simulink model "sampleModel1488"  (R2023a)
settings: Solver=VariableStepAuto  StartTime=0.0  StopTime=10.0  RelTol=1e-3
undefined symbols (not defined in the file): b011101a, b0c8, bf87616c, DiscIntNeverNeededParam, Newton, Raphson
libraries: simulink x171, slpidlib x32, simulink_need_slupdate x2
(part 5 of 6)

== system sampleModel1488/cfblk153/cfblk12 ==
  cfblk1 : Inport
  cfblk9 : Inport  Port=2
  cfblk11 : Delay  SampleTime=1
  cfblk12 : Delay  SampleTime=1
  cfblk3 : DiscreteFilter  SampleTime=1
  cfblk4 : Gain  Gain=[185491925.881963]
  cfblk5 : Product
  cfblk6 : ComplexToMagnitudeAngle
  cfblk7 : MinMax  Inputs=3
  cfblk8 : simulink/Math Operations/Slider Gain  gain=1  low=0  high=2
  cfblk2 : Outport
  cfblk10 : Outport  Port=2
  wires:
  cfblk9/1 -> cfblk8/1
  cfblk3/1 -> cfblk6/1
  cfblk7/1 -> cfblk2/1, cfblk3/1
  cfblk8/1 -> cfblk4/1
  cfblk5/1 -> cfblk7/2
  cfblk1/1 -> cfblk5/1, cfblk7/3
  cfblk4/1 -> cfblk10/1
  cfblk6/1 -> cfblk11/1
  cfblk11/1 -> cfblk7/1
  cfblk6/2 -> cfblk12/1
  cfblk12/1 -> cfblk5/2

== system sampleModel1488/cfblk153/cfblk8 ==
  cfblk1 : Inport
  cfblk9 : Inport  Port=2
  cfblk3 : DiscreteTransferFcn  SampleTime=1
  cfblk4 : simulink/Discrete/Transfer Fcn First Order  PoleZ=0.95  ICPrevOutput=0.0  DoSatur=off
  cfblk5 : simulink/Discrete/Transfer Fcn Lead or Lag  PoleZ=0.95  ZeroZ=0.75  ICPrevOutput=0.0  ICPrevInput=0.0  DoSatur=off
  cfblk6 : ComplexToRealImag
  cfblk7 : Product  Inputs=**
  cfblk8 : Constant  Value=[-545162540.511820]  SampleTime=1
  cfblk2 : Outport
  cfblk10 : Outport  Port=2
  wires:
  cfblk1/1 -> cfblk5/1
  cfblk5/1 -> cfblk2/1
  cfblk7/1 -> cfblk4/1
  cfblk3/1 -> cfblk6/1
  cfblk6/1 -> cfblk7/1
  cfblk8/1 -> cfblk7/2
  cfblk9/1 -> cfblk3/1
  cfblk4/1 -> cfblk10/1

== system sampleModel1488/cfblk153/cfblk9 ==
  cfblk1 : Inport
  cfblk7 : Inport  Port=2
  cfblk3 : DiscreteZeroPole  Poles=[0 0.5]  Gain=1
  cfblk4 : Bias  Bias=[67062085.652409]  SaturateOnIntegerOverflow=off
  cfblk5 : ComplexToRealImag
  cfblk6 : Rounding
  cfblk9 : Delay  SampleTime=1
  cfblk2 : Outport
  cfblk8 : Outport  Port=2
  wires:
  cfblk3/1 -> cfblk6/1
  cfblk5/1 -> cfblk8/1
  cfblk5/2 -> cfblk2/1
  cfblk1/1 -> cfblk5/1
  cfblk7/1 -> cfblk4/1
  cfblk6/1 -> cfblk9/1
  cfblk9/1 -> cfblk3/1

== system sampleModel1488/cfblk154/cfblk7 ==
  cfblk1 : Inport
  cfblk6 : Inport  Port=2
  cfblk3 : Delay  ShowEnablePort=on  SampleTime=1
      settings: InputPortMap=u0,e6
  cfblk4 : simulink/Discrete/Difference  ICPrevInput=0.0  OutMin=[]  OutMax=[]  OutDataTypeStr=Inherit: Inherit via back propagation  OutDataType=fixdt(1, 16)  OutScaling=2^-10  DoSatur=off
  cfblk5 : Rounding
  cfblk2 : Outport
  cfblk7 : Outport  Port=2
  wires:
  cfblk3/1 -> cfblk7/1
  cfblk1/1 -> cfblk2/1
  cfblk4/1 -> cfblk3/1
  cfblk6/1 -> cfblk5/1, cfblk3/2
  cfblk5/1 -> cfblk4/1

== system sampleModel1488/cfblk155/cfblk5 ==
  cfblk1 : Inport
  cfblk12 : Inport  Port=2
  cfblk13 : Inport  Port=3
  cfblk14 : Inport  Port=4
  cfblk10 : Constant  Value=[300138344.882590]  SampleTime=1
  cfblk11 : Constant  Value=[340060627.789807]  SampleTime=1
  cfblk3 : DiscreteIntegrator  ICPrevOutput=DiscIntNeverNeededParam  ICPrevScaledInput=DiscIntNeverNeededParam
  cfblk4 : DiscreteFilter  SampleTime=1
  cfblk5 : simulink/Discrete/Tapped Delay  vinit=0.0  samptime=-1  NumDelays=1  DelayOrder=Oldest  includeCurrent=off
  cfblk6 : UnaryMinus
  cfblk7 : DotProduct  OutDataTypeStr=Inherit: Inherit via internal rule
  cfblk8 : DotProduct  OutDataTypeStr=Inherit: Inherit via internal rule
  cfblk9 : Squeeze
  cfblk2 : Outport
  cfblk15 : Outport  Port=2
  wires:
  cfblk8/1 -> cfblk3/1
  cfblk4/1 -> cfblk2/1
  cfblk10/1 -> cfblk7/1
  cfblk3/1 -> cfblk7/2
  cfblk5/1 -> cfblk8/1
  cfblk1/1 -> cfblk5/1
  cfblk11/1 -> cfblk6/1
  cfblk14/1 -> cfblk9/1
  cfblk13/1 -> cfblk8/2
  cfblk9/1 -> cfblk4/1
  cfblk7/1 -> cfblk15/1

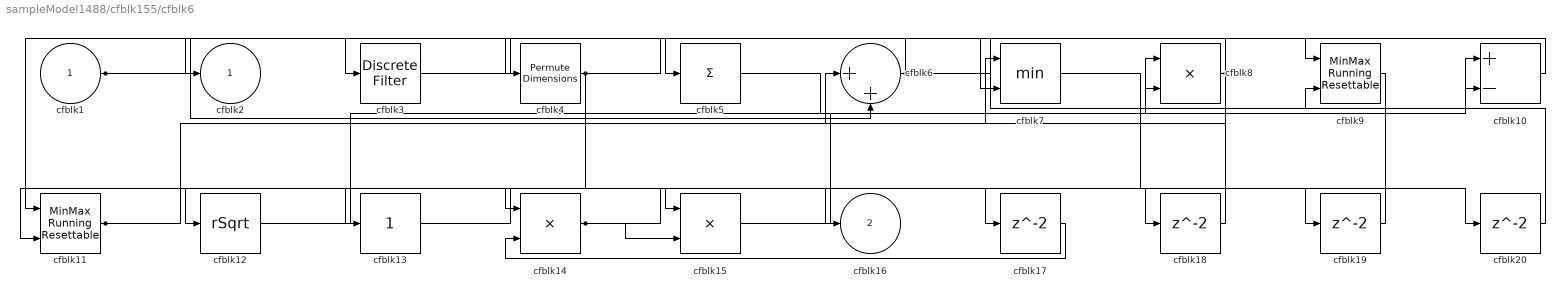
== system sampleModel1488/cfblk155/cfblk6 ==
  cfblk1 : Inport
  cfblk10 : Sum  Inputs=+-
  cfblk11 : simulink/Math Operations/MinMax Running Resettable  Function=min  vinit=0.0
  cfblk12 : Sqrt  Operator=rSqrt  AlgorithmType=Newton-Raphson
  cfblk13 : simulink/Math Operations/Slider Gain  gain=1  low=0  high=2
  cfblk14 : Product
  cfblk15 : Product  Inputs=**
  cfblk{17..20} (4 alike) : Delay  SampleTime=1
  cfblk3 : DiscreteFilter  SampleTime=1
  cfblk4 : PermuteDimensions
  cfblk5 : Sum  Inputs=+
  cfblk6 : Sum  Inputs=|++
  cfblk7 : MinMax  Inputs=2
  cfblk8 : Product
  cfblk9 : simulink/Math Operations/MinMax Running Resettable  Function=min  vinit=0.0
  cfblk2 : Outport
  cfblk16 : Outport  Port=2
  wires:
  cfblk4/1 -> cfblk12/1, cfblk7/2
  cfblk10/1 -> cfblk11/1
  cfblk3/1 -> cfblk5/1
  cfblk15/1 -> cfblk8/1
  cfblk11/1 -> cfblk7/1, cfblk13/1, cfblk18/1
  cfblk13/1 -> cfblk16/1
  cfblk12/1 -> cfblk10/1
  cfblk9/1 -> cfblk14/1
  cfblk5/1 -> cfblk8/2
  cfblk6/1 -> cfblk9/1, cfblk3/1, cfblk10/2
  cfblk8/1 -> cfblk11/2, cfblk2/1, cfblk17/1
  cfblk14/1 -> cfblk15/2, cfblk20/1
  cfblk1/1 -> cfblk6/2, cfblk4/1
  cfblk17/1 -> cfblk14/2
  cfblk18/1 -> cfblk6/1
  cfblk7/1 -> cfblk19/1
  cfblk19/1 -> cfblk15/1
  cfblk20/1 -> cfblk9/2

== system sampleModel1488/cfblk156/cfblk10 ==
  cfblk1 : Inport
  cfblk10 : Inport  Port=2
  cfblk11 : Inport  Port=3
  cfblk12 : Inport  Port=4
  cfblk13 : Inport  Port=5
  cfblk14 : Inport  Port=6
  cfblk15 : Inport  Port=7
  cfblk3 : simulink/Discrete/Transfer Fcn Real Zero  ZeroZ=0.75  ICPrevInput=0.0  DoSatur=off
  cfblk4 : Delay  DelayLengthSource=Input port  SampleTime=1
      settings: InputPortMap=u0,p1
  cfblk5 : simulink/Math Operations/MinMax Running Resettable  Function=min  vinit=0.0
  cfblk6 : UnaryMinus
  cfblk7 : Squeeze
  cfblk8 : Rounding
  cfblk9 : Constant  Value=[895322643.811582]  SampleTime=1
  cfblk2 : Outport
  wires:
  cfblk10/1 -> cfblk4/1
  cfblk5/1 -> cfblk2/1
  cfblk3/1 -> cfblk6/1
  cfblk1/1 -> cfblk5/1
  cfblk13/1 -> cfblk4/2
  cfblk8/1 -> cfblk5/2
  cfblk7/1 -> cfblk8/1
  cfblk11/1 -> cfblk7/1
  cfblk15/1 -> cfblk3/1

== system sampleModel1488/cfblk156/cfblk11 ==
  cfblk1 : Inport
  cfblk6 : Inport  Port=2
  cfblk7 : Inport  Port=3
  cfblk8 : Inport  Port=4
  cfblk9 : Inport  Port=5
  cfblk3 : Product  Inputs=*
  cfblk4 : Squeeze
  cfblk5 : Constant  Value=[-712808178.157730]  SampleTime=1
  cfblk2 : Outport
  cfblk10 : Outport  Port=2
  wires:
  cfblk6/1 -> cfblk2/1
  cfblk1/1 -> cfblk4/1
  cfblk8/1 -> cfblk10/1
  cfblk4/1 -> cfblk3/1

== system sampleModel1488/cfblk156/cfblk12 ==
  cfblk1 : Inport
  cfblk9 : Inport  Port=2
  cfblk10 : Inport  Port=3
  cfblk11 : Inport  Port=4
  cfblk3 : simulink/Discrete/Transfer Fcn Lead or Lag  PoleZ=0.95  ZeroZ=0.75  ICPrevOutput=0.0  ICPrevInput=0.0  DoSatur=off
  cfblk4 : Bias  Bias=[-19724596.447759]  SaturateOnIntegerOverflow=off
  cfblk5 : Abs  SaturateOnIntegerOverflow=off
  cfblk6 : Product
  cfblk7 : Assignment  DiagnosticForDimensions=Warning  IndexOptions=Index vector (dialog)  Indices=1  OutputSizes=1
  cfblk8 : Constant  Value=[-371159435.516197]  SampleTime=1
  cfblk2 : Outport
  wires:
  cfblk6/1 -> cfblk7/1
  cfblk10/1 -> cfblk5/1
  cfblk9/1 -> cfblk3/1
  cfblk3/1 -> cfblk4/1
  cfblk4/1 -> cfblk6/1
  cfblk7/1 -> cfblk2/1
  cfblk11/1 -> cfblk6/2
  cfblk1/1 -> cfblk7/2

== system sampleModel1488/cfblk157/cfblk12 ==
  cfblk1 : Inport
  cfblk5 : Inport  Port=2
  cfblk6 : Inport  Port=3
  cfblk7 : Inport  Port=4
  cfblk8 : Inport  Port=5
  Action Port : ActionPort  ActionPortLabel=if(u1 >= 0)
  cfblk3 : Product
  cfblk4 : ComplexToMagnitudeAngle
  cfblk2 : Outport
  wires:
  cfblk5/1 -> cfblk4/1
  cfblk1/1 -> cfblk2/1
  cfblk6/1 -> cfblk3/1
  cfblk4/1 -> cfblk3/2

== system sampleModel1488/cfblk157/cfblk13 ==
  cfblk1 : Inport
  cfblk11 : Inport  Port=2
  cfblk12 : Inport  Port=3
  cfblk13 : Inport  Port=4
  Action Port : ActionPort  ActionPortLabel=else
  cfblk10 : Constant  Value=[-560694397.866348]  SampleTime=1
  cfblk3 : simulink/Discrete/Tapped Delay  vinit=0.0  samptime=-1  NumDelays=1  DelayOrder=Oldest  includeCurrent=off
  cfblk4 : simulink/Discrete/Transfer Fcn Real Zero  ZeroZ=0.75  ICPrevInput=0.0  DoSatur=off
  cfblk5 : UnaryMinus
  cfblk6 : Signum
  cfblk7 : Signum
  cfblk8 : Gain  Gain=[983882556.458164]
  cfblk9 : Constant  Value=[-401635952.431954]  SampleTime=1
  cfblk2 : Outport
  cfblk14 : Outport  Port=2
  cfblk15 : Outport  Port=3
  cfblk16 : Outport  Port=4
  wires:
  cfblk11/1 -> cfblk6/1
  cfblk10/1 -> cfblk5/1
  cfblk6/1 -> cfblk14/1
  cfblk7/1 -> cfblk8/1
  cfblk5/1 -> cfblk16/1
  cfblk13/1 -> cfblk7/1
  cfblk8/1 -> cfblk3/1
  cfblk1/1 -> cfblk2/1
  cfblk3/1 -> cfblk15/1
  cfblk12/1 -> cfblk4/1

== system sampleModel1488/cfblk158/cfblk11 ==
  cfblk1 : Inport
  cfblk15 : Inport  Port=2
  cfblk16 : Inport  Port=3
  cfblk17 : Inport  Port=4
  cfblk10 : UnaryMinus
  cfblk11 : Product  Inputs=*
  cfblk12 : Constant  Value=[-127465425.334475]  SampleTime=1
  cfblk13 : Constant  Value=[-255537626.018522]  SampleTime=1
  cfblk14 : Constant  Value=[421184774.119450]  SampleTime=1
  cfblk3 : DiscreteStateSpace
  cfblk4 : Abs  SaturateOnIntegerOverflow=off
  cfblk5 : Sum  Inputs=+
  cfblk6 : Squeeze
  cfblk7 : Product  Inputs=*
  cfblk8 : Bias  Bias=[52580442.536765]  SaturateOnIntegerOverflow=off
  cfblk9 : Sum  Inputs=|++
  cfblk2 : Outport
  wires:
  cfblk12/1 -> cfblk5/1
  cfblk16/1 -> cfblk11/1
  cfblk1/1 -> cfblk6/1
  cfblk14/1 -> cfblk9/1
  cfblk8/1 -> cfblk2/1
  cfblk6/1 -> cfblk4/1
  cfblk9/1 -> cfblk8/1
  cfblk13/1 -> cfblk10/1
  cfblk11/1 -> cfblk3/1
  cfblk10/1 -> cfblk9/2
  cfblk5/1 -> cfblk7/1

== system sampleModel1488/cfblk158/cfblk12 ==
  cfblk1 : Inport
  cfblk10 : Constant  Value=[-764079549.209031]  SampleTime=1
  cfblk11 : Delay  SampleTime=1
  cfblk12 : Delay  SampleTime=1
  cfblk3 : simulink/Discrete/Tapped Delay  vinit=0.0  samptime=-1  NumDelays=1  DelayOrder=Oldest  includeCurrent=off
  cfblk4 : DiscreteStateSpace
  cfblk5 : Sqrt  Operator=rSqrt  AlgorithmType=Newton-Raphson
  cfblk6 : Bias  Bias=[-61616886.932109]  SaturateOnIntegerOverflow=off
  cfblk7 : Sum  Inputs=+-
  cfblk8 : Polyval  Coefs=[ +2.081618890e-019, -1.441693666e-014, +4.719686976e-010, -8.536869453e-006, +1.621573104e-001, -8.087801117e+001 ]
  cfblk9 : Gain  Gain=[-336532196.951205]
  cfblk2 : Outport
  wires:
  cfblk5/1 -> cfblk6/1
  cfblk9/1 -> cfblk4/1
  cfblk7/1 -> cfblk8/1
  cfblk4/1 -> cfblk7/1
  cfblk1/1 -> cfblk9/1
  cfblk3/1 -> cfblk2/1
  cfblk10/1 -> cfblk3/1
  cfblk8/1 -> cfblk11/1
  cfblk11/1 -> cfblk7/2
  cfblk6/1 -> cfblk12/1
  cfblk12/1 -> cfblk5/1

== system sampleModel1488/cfblk159/cfblk10 ==
  cfblk1 : Inport
  cfblk7 : Inport  Port=2
  cfblk3 : DiscreteZeroPole  Poles=[0 0.5]  Gain=1
  cfblk4 : slpidlib/PID Controller  Controller=PID  Form=Parallel  TimeDomain=Discrete-time  UseExternalTs=off  SampleTime=1  IntegratorMethod=Forward Euler  FilterMethod=Forward Euler  ControllerParametersSource=internal  P=1  I=1  UseKiTs=off  D=0  N=100  UseFilter=on  TunerSelectOption=Transfer Function Based (PID Tuner App)  InitialConditionSource=internal  InitialConditionForIntegrator=0  InitialConditionForFilter=0  DifferentiatorICPrevScaledInput=0  ExternalReset=none  TrackingMode=off  Kt=1  LimitOutput=off  SatLimitsSource=internal  UpperSaturationLimit=inf  LowerSaturationLimit=-inf  LinearizeAsGain=off  AntiWindupMode=none  Kb=1  LimitIntegrator=off  UpperIntegratorSaturationLimit=inf  LowerIntegratorSaturationLimit=-inf  POutMin=[]  POutMax=[]  IOutMin=[]  IOutMax=[]  DOutMin=[]  DOutMax=[]  NOutMin=[]  NOutMax=[]  SumOutMin=[]  SumOutMax=[]  SaturationOutMin=[]  SaturationOutMax=[]  PParamMin=[]  PParamMax=[]  IParamMin=[]  IParamMax=[]  DParamMin=[]  DParamMax=[]  NParamMin=[]  NParamMax=[]  KbParamMin=[]  KbParamMax=[]  KtParamMin=[]  KtParamMax=[]  KbOutMin=[]  KbOutMax=[]  KtOutMin=[]  KtOutMax=[]  IntegratorOutMin=[]  IntegratorOutMax=[]  FilterOutMin=[]  FilterOutMax=[]  SumI1OutMin=[]  SumI1OutMax=[]  SumI2OutMin=[]  SumI2OutMax=[]  SumI3OutMin=[]  SumI3OutMax=[]  SumI4OutMin=[]  SumI4OutMax=[]  SumDOutMin=[]  SumDOutMax=[]  DifferentiatorOutMin=[]  DifferentiatorOutMax=[]  FilterDiffOutCoefMin=[]  FilterDiffOutCoefMax=[]  ReciprocalOutMin=[]  ReciprocalOutMax=[]  SumDenOutMin=[]  SumDenOutMax=[]  SumNumOutMin=[]  SumNumOutMax=[]  DivideOutMin=[]  DivideOutMax=[]  UdiffTsProdOutMin=[]  UdiffTsProdOutMax=[]  NTsProdOutMin=[]  NTsProdOutMax=[]  UintegralTsProdOutMin=[]  UintegralTsProdOutMax=[]  UngainTsProdOutMin=[]  UngainTsProdOutMax=[]  ClampingZeroOutDataTypeStr=Inherit: Inherit via back propagation  ClampingZeroOutMin=[]  ClampingZeroOutMax=[]  FilterDenConstantOutDataTypeStr=Inherit: Inherit via back propagation  FilterDenConstantOutMin=[]  FilterDenConstantOutMax=[]  PCopyOutDataTypeStr=Inherit: Inherit via back propagation  PCopyOutMin=[]  PCopyOutMax=[]  NCopyOutDataTypeStr=Inherit: Inherit via back propagation  NCopyOutMin=[]  NCopyOutMax=[]  IntegratorContinuousStateAttributes=''  IntegratorStateMustResolveToSignalObject=off  IntegratorRTWStateStorageClass=Auto  FilterContinuousStateAttributes=''  FilterStateMustResolveToSignalObject=off  FilterRTWStateStorageClass=Auto  ParallelPVariant=InternalParameters  IdealPVariant=Disabled  IVariant=InternalParameters  DVariant=InternalParameters  IntegratorVariant=Discrete  SatVariant=Disabled  AWVariant=Passthrough  PCopyVariant=Disabled  TRVariant=Disabled  FdbkBlocksVariant=Forward  IdealPFdbkVariant=Disabled  SatFdbkVariant=Disabled  DerivativeFilterVariant=ForwardEulerFilter  NVariant=InternalParameters  NCopyVariant=Disabled  FilterICVariant=InternalICsFilter  IntegratorICVariant=InternalICs  ExternalResetVariant=Disabled  TRSumVariant=Passthrough  SumFdbkVariant=Disabled  SumVariant=Sum_PID  TsampFilterVariant=InternalTs  TsampNgainVariant=Passthrough  TsampIntegralVariant=Disabled_SignalSpec  ExternalSaturationOutDataTypeStr=Inherit: Same as second input
      settings: LibrarySourceBlock=simulink/Discrete/Discrete PID Controller
  cfblk5 : DiscreteTransferFcn  SampleTime=1
  cfblk6 : UnaryMinus
  cfblk2 : Outport
  wires:
  cfblk3/1 -> cfblk2/1
  cfblk1/1 -> cfblk3/1
  cfblk7/1 -> cfblk4/1
  cfblk4/1 -> cfblk5/1
  cfblk5/1 -> cfblk6/1

== system sampleModel1488/cfblk159/cfblk13 ==
  cfblk1 : Inport
  cfblk13 : Inport  Port=2
  cfblk14 : Inport  Port=3
  cfblk15 : Inport  Port=4
  Action Port : ActionPort  ActionPortLabel=if(u1 >= 0)
  cfblk10 : Constant  Value=[445844629.923576]  SampleTime=1
  cfblk11 : Constant  Value=[-767676782.462914]  SampleTime=1
  cfblk12 : Constant  Value=[-250313650.922789]  SampleTime=1
  cfblk3 : simulink/Discrete/Tapped Delay  vinit=0.0  samptime=-1  NumDelays=1  DelayOrder=Oldest  includeCurrent=off
  cfblk4 : DiscreteFilter
  cfblk5 : simulink/Math Operations/MinMax Running Resettable  Function=min  vinit=0.0
  cfblk6 : Sqrt
  cfblk7 : PermuteDimensions
  cfblk8 : Sqrt  Operator=rSqrt  AlgorithmType=Newton-Raphson
  cfblk9 : Sum  Inputs=+-
  cfblk2 : Outport
  wires:
  cfblk11/1 -> cfblk7/1
  cfblk9/1 -> cfblk3/1
  cfblk6/1 -> cfblk4/1
  cfblk12/1 -> cfblk5/1
  cfblk3/1 -> cfblk6/1
  cfblk10/1 -> cfblk2/1
  cfblk4/1 -> cfblk8/1
  cfblk1/1 -> cfblk5/2
  cfblk7/1 -> cfblk9/1
  cfblk13/1 -> cfblk9/2

== system sampleModel1488/cfblk159/cfblk14 ==
  cfblk1 : Inport
  cfblk9 : Inport  Port=2
  Action Port : ActionPort  ActionPortLabel=else
  cfblk10 : Delay
  cfblk3 : DiscreteStateSpace  SampleTime=-1
  cfblk4 : Bias  Bias=[827812875.693291]  SaturateOnIntegerOverflow=off
  cfblk5 : MinMax  Function=max
  cfblk6 : Sum  Inputs=--
  cfblk7 : Squeeze
  cfblk8 : Product  Inputs=**
  cfblk2 : Outport
  wires:
  cfblk6/1 -> cfblk2/1
  cfblk4/1 -> cfblk5/1
  cfblk9/1 -> cfblk7/1
  cfblk7/1 -> cfblk4/1
  cfblk1/1 -> cfblk8/2, cfblk6/2
  cfblk5/1 -> cfblk6/1
  cfblk8/1 -> cfblk3/1
  cfblk3/1 -> cfblk10/1
  cfblk10/1 -> cfblk8/1

== system sampleModel1488/cfblk159/cfblk7 ==
  cfblk1 : Inport
  cfblk10 : Inport  Port=2
  cfblk13 : Delay  SampleTime=1
  cfblk3 : simulink/Discrete/Transfer Fcn First Order  PoleZ=0.95  ICPrevOutput=0.0  DoSatur=off
  cfblk4 : Signum
  cfblk5 : Gain  Gain=[678568450.449569]
  cfblk6 : Gain  Gain=[-280068207.305147]
  cfblk7 : Sum  Inputs=+-
  cfblk8 : DotProduct  OutDataTypeStr=Inherit: Inherit via internal rule
  cfblk9 : Trigonometry
  cfblk2 : Outport
  cfblk11 : Outport  Port=2
  cfblk12 : Outport  Port=3
  wires:
  cfblk5/1 -> cfblk7/1
  cfblk9/1 -> cfblk3/1, cfblk11/1
  cfblk4/1 -> cfblk12/1
  cfblk8/1 -> cfblk6/1
  cfblk3/1 -> cfblk8/2
  cfblk7/1 -> cfblk9/1, cfblk4/1
  cfblk1/1 -> cfblk2/1, cfblk5/1
  cfblk10/1 -> cfblk7/2
  cfblk6/1 -> cfblk13/1
  cfblk13/1 -> cfblk8/1

== system sampleModel1488/cfblk159/cfblk8 ==
  cfblk1 : Inport
  cfblk6 : Inport  Port=2
  cfblk7 : Inport  Port=3
  cfblk8 : Inport  Port=4
  cfblk3 : simulink/Math Operations/Slider Gain  gain=1  low=0  high=2
  cfblk4 : Reshape
  cfblk5 : Assignment  DiagnosticForDimensions=Warning  IndexOptions=Index vector (dialog)  Indices=1  OutputSizes=1
  cfblk2 : Outport
  wires:
  cfblk6/1 -> cfblk5/1
  cfblk4/1 -> cfblk3/1
  cfblk7/1 -> cfblk4/1
  cfblk3/1 -> cfblk5/2
  cfblk1/1 -> cfblk2/1

== system sampleModel1488/cfblk159/cfblk9 ==
  cfblk1 : Inport
  cfblk7 : Inport  Port=2
  cfblk8 : Inport  Port=3
  cfblk9 : Inport  Port=4
  cfblk10 : Inport  Port=5
  cfblk3 : simulink/Discrete/Tapped Delay  vinit=0.0  samptime=-1  NumDelays=1  DelayOrder=Oldest  includeCurrent=off
  cfblk4 : Delay  ShowEnablePort=on  SampleTime=1
      settings: InputPortMap=u0,e6
  cfblk5 : MinMax  Function=max
  cfblk6 : ComplexToRealImag
  cfblk2 : Outport
  wires:
  cfblk10/1 -> cfblk3/1
  cfblk5/1 -> cfblk6/1
  cfblk8/1 -> cfblk2/1
  cfblk9/1 -> cfblk5/1
  cfblk7/1 -> cfblk4/1
  cfblk1/1 -> cfblk4/2

== system sampleModel1488/cfblk160/cfblk10 ==
  cfblk1 : Inport
  cfblk8 : Inport  Port=2
  cfblk10 : Delay  SampleTime=1
  cfblk3 : simulink/Discrete/Transfer Fcn Lead or Lag  PoleZ=0.95  ZeroZ=0.75  ICPrevOutput=0.0  ICPrevInput=0.0  DoSatur=off
  cfblk4 : Gain  Gain=[940902474.702372]
  cfblk5 : Sum  Inputs=+-
  cfblk6 : Sum  Inputs=+
  cfblk7 : Reshape
  cfblk9 : Delay  SampleTime=1
  cfblk2 : Outport
  wires:
  cfblk4/1 -> cfblk5/1
  cfblk1/1 -> cfblk2/1
  cfblk7/1 -> cfblk5/2
  cfblk8/1 -> cfblk7/1
  cfblk3/1 -> cfblk6/1
  cfblk6/1 -> cfblk9/1
  cfblk9/1 -> cfblk3/1
  cfblk5/1 -> cfblk10/1
  cfblk10/1 -> cfblk4/1

== system sampleModel1488/cfblk160/cfblk11 ==
  cfblk1 : Inport
  cfblk15 : Inport  Port=2
  cfblk10 : MinMax  Function=max  Inputs=3
  cfblk11 : Reshape
  cfblk12 : DotProduct  OutDataTypeStr=Inherit: Inherit via internal rule
  cfblk13 : Constant  Value=[806111497.485991]  SampleTime=1
  cfblk14 : Constant  Value=[673108402.113874]  SampleTime=1
  cfblk3 : DiscreteStateSpace
  cfblk4 : Delay  ShowEnablePort=on  SampleTime=1
      settings: InputPortMap=u0,e6
  cfblk5 : simulink/Discrete/Tapped Delay  vinit=0.0  samptime=-1  NumDelays=1  DelayOrder=Oldest  includeCurrent=off
  cfblk6 : DiscreteIntegrator  ICPrevOutput=DiscIntNeverNeededParam  ICPrevScaledInput=DiscIntNeverNeededParam
  cfblk7 : DiscreteTransferFcn  SampleTime=1
  cfblk8 : Rounding
  cfblk9 : Bias  Bias=[917586938.243166]  SaturateOnIntegerOverflow=off
  cfblk2 : Outport
  wires:
  cfblk7/1 -> cfblk12/1
  cfblk5/1 -> cfblk6/1
  cfblk15/1 -> cfblk12/2
  cfblk12/1 -> cfblk5/1
  cfblk10/1 -> cfblk4/1
  cfblk8/1 -> cfblk4/2
  cfblk4/1 -> cfblk7/1
  cfblk3/1 -> cfblk11/1
  cfblk1/1 -> cfblk8/1
  cfblk13/1 -> cfblk10/1
  cfblk14/1 -> cfblk10/2, cfblk3/1
  cfblk9/1 -> cfblk10/3
  cfblk11/1 -> cfblk9/1
  cfblk6/1 -> cfblk2/1

== system sampleModel1488/cfblk160/cfblk6 ==
  cfblk1 : Inport
  cfblk8 : Inport  Port=2
  cfblk9 : Inport  Port=3
  cfblk10 : Inport  Port=4
  cfblk3 : Rounding
  cfblk4 : Sum  Inputs=|++
  cfblk5 : Rounding
  cfblk6 : Sum
  cfblk7 : Squeeze
  cfblk2 : Outport
  cfblk11 : Outport  Port=2
  cfblk12 : Outport  Port=3
  wires:
  cfblk9/1 -> cfblk5/1
  cfblk1/1 -> cfblk4/1
  cfblk8/1 -> cfblk7/1
  cfblk10/1 -> cfblk3/1
  cfblk4/1 -> cfblk11/1
  cfblk6/1 -> cfblk12/1
  cfblk5/1 -> cfblk2/1
  cfblk3/1 -> cfblk4/2
  cfblk7/1 -> cfblk6/1, cfblk6/2

== system sampleModel1488/cfblk160/cfblk7 ==
  cfblk1 : Inport
  cfblk13 : Inport  Port=2
  cfblk14 : Inport  Port=3
  cfblk10 : Constant  Value=[187633788.558614]  SampleTime=1
  cfblk11 : Constant  Value=[646595502.135629]  SampleTime=1
  cfblk12 : Constant  Value=[-119798684.754510]  SampleTime=1
  cfblk15 : Delay  SampleTime=1
  cfblk16 : Delay  SampleTime=1
  cfblk3 : simulink/Discrete/Difference  ICPrevInput=0.0  OutMin=[]  OutMax=[]  OutDataTypeStr=Inherit: Inherit via back propagation  OutDataType=fixdt(1, 16)  OutScaling=2^-10  DoSatur=off
  cfblk4 : simulink/Discrete/Transfer Fcn First Order  PoleZ=0.95  ICPrevOutput=0.0  DoSatur=off
  cfblk5 : Sum  Inputs=+-
  cfblk6 : DotProduct  OutDataTypeStr=Inherit: Inherit via internal rule
  cfblk7 : MinMax  Function=max  Inputs=3
  cfblk8 : UnaryMinus
  cfblk9 : Sum  Inputs=|++
  cfblk2 : Outport
  wires:
  cfblk3/1 -> cfblk8/1
  cfblk11/1 -> cfblk2/1
  cfblk13/1 -> cfblk7/1, cfblk6/2
  cfblk1/1 -> cfblk5/1
  cfblk12/1 -> cfblk5/2
  cfblk14/1 -> cfblk6/1
  cfblk5/1 -> cfblk9/1
  cfblk10/1 -> cfblk4/1
  cfblk4/1 -> cfblk7/2
  cfblk9/1 -> cfblk7/3
  cfblk7/1 -> cfblk15/1
  cfblk15/1 -> cfblk9/2
  cfblk8/1 -> cfblk16/1
  cfblk16/1 -> cfblk3/1

== system sampleModel1488/cfblk160/cfblk8 ==
  cfblk1 : Inport
  cfblk12 : Inport  Port=2
  cfblk13 : Inport  Port=3
  cfblk14 : Inport  Port=4
  cfblk10 : Constant  Value=[-873178605.065547]  SampleTime=1
  cfblk11 : Constant  Value=[-412309283.831914]  SampleTime=1
  cfblk3 : slpidlib/PID Controller  Controller=PID  Form=Parallel  TimeDomain=Discrete-time  UseExternalTs=off  SampleTime=1  IntegratorMethod=Forward Euler  FilterMethod=Forward Euler  ControllerParametersSource=internal  P=1  I=1  UseKiTs=off  D=0  N=100  UseFilter=on  TunerSelectOption=Transfer Function Based (PID Tuner App)  InitialConditionSource=internal  InitialConditionForIntegrator=0  InitialConditionForFilter=0  DifferentiatorICPrevScaledInput=0  ExternalReset=none  TrackingMode=off  Kt=1  LimitOutput=off  SatLimitsSource=internal  UpperSaturationLimit=inf  LowerSaturationLimit=-inf  LinearizeAsGain=off  AntiWindupMode=none  Kb=1  LimitIntegrator=off  UpperIntegratorSaturationLimit=inf  LowerIntegratorSaturationLimit=-inf  POutMin=[]  POutMax=[]  IOutMin=[]  IOutMax=[]  DOutMin=[]  DOutMax=[]  NOutMin=[]  NOutMax=[]  SumOutMin=[]  SumOutMax=[]  SaturationOutMin=[]  SaturationOutMax=[]  PParamMin=[]  PParamMax=[]  IParamMin=[]  IParamMax=[]  DParamMin=[]  DParamMax=[]  NParamMin=[]  NParamMax=[]  KbParamMin=[]  KbParamMax=[]  KtParamMin=[]  KtParamMax=[]  KbOutMin=[]  KbOutMax=[]  KtOutMin=[]  KtOutMax=[]  IntegratorOutMin=[]  IntegratorOutMax=[]  FilterOutMin=[]  FilterOutMax=[]  SumI1OutMin=[]  SumI1OutMax=[]  SumI2OutMin=[]  SumI2OutMax=[]  SumI3OutMin=[]  SumI3OutMax=[]  SumI4OutMin=[]  SumI4OutMax=[]  SumDOutMin=[]  SumDOutMax=[]  DifferentiatorOutMin=[]  DifferentiatorOutMax=[]  FilterDiffOutCoefMin=[]  FilterDiffOutCoefMax=[]  ReciprocalOutMin=[]  ReciprocalOutMax=[]  SumDenOutMin=[]  SumDenOutMax=[]  SumNumOutMin=[]  SumNumOutMax=[]  DivideOutMin=[]  DivideOutMax=[]  UdiffTsProdOutMin=[]  UdiffTsProdOutMax=[]  NTsProdOutMin=[]  NTsProdOutMax=[]  UintegralTsProdOutMin=[]  UintegralTsProdOutMax=[]  UngainTsProdOutMin=[]  UngainTsProdOutMax=[]  ClampingZeroOutDataTypeStr=Inherit: Inherit via back propagation  ClampingZeroOutMin=[]  ClampingZeroOutMax=[]  FilterDenConstantOutDataTypeStr=Inherit: Inherit via back propagation  FilterDenConstantOutMin=[]  FilterDenConstantOutMax=[]  PCopyOutDataTypeStr=Inherit: Inherit via back propagation  PCopyOutMin=[]  PCopyOutMax=[]  NCopyOutDataTypeStr=Inherit: Inherit via back propagation  NCopyOutMin=[]  NCopyOutMax=[]  IntegratorContinuousStateAttributes=''  IntegratorStateMustResolveToSignalObject=off  IntegratorRTWStateStorageClass=Auto  FilterContinuousStateAttributes=''  FilterStateMustResolveToSignalObject=off  FilterRTWStateStorageClass=Auto  ParallelPVariant=InternalParameters  IdealPVariant=Disabled  IVariant=InternalParameters  DVariant=InternalParameters  IntegratorVariant=Discrete  SatVariant=Disabled  AWVariant=Passthrough  PCopyVariant=Disabled  TRVariant=Disabled  FdbkBlocksVariant=Forward  IdealPFdbkVariant=Disabled  SatFdbkVariant=Disabled  DerivativeFilterVariant=ForwardEulerFilter  NVariant=InternalParameters  NCopyVariant=Disabled  FilterICVariant=InternalICsFilter  IntegratorICVariant=InternalICs  ExternalResetVariant=Disabled  TRSumVariant=Passthrough  SumFdbkVariant=Disabled  SumVariant=Sum_PID  TsampFilterVariant=InternalTs  TsampNgainVariant=Passthrough  TsampIntegralVariant=Disabled_SignalSpec  ExternalSaturationOutDataTypeStr=Inherit: Same as second input
      settings: LibrarySourceBlock=simulink/Discrete/Discrete PID Controller
  cfblk4 : DiscreteZeroPole  Poles=[0 0.5]  Gain=1
  cfblk5 : simulink/Math Operations/MinMax Running Resettable  Function=min  vinit=0.0
  cfblk6 : Abs  SaturateOnIntegerOverflow=off
  cfblk7 : Product  Inputs=**
  cfblk8 : Sqrt  Operator=rSqrt  AlgorithmType=Newton-Raphson
  cfblk9 : Constant  Value=[-794780800.463545]  SampleTime=1
  cfblk2 : Outport
  cfblk15 : Outport  Port=2
  cfblk16 : Outport  Port=3
  cfblk17 : Outport  Port=4
  wires:
  cfblk6/1 -> cfblk5/1
  cfblk11/1 -> cfblk16/1
  cfblk9/1 -> cfblk3/1
  cfblk5/1 -> cfblk15/1
  cfblk12/1 -> cfblk17/1
  cfblk13/1 -> cfblk5/2
  cfblk14/1 -> cfblk6/1
  cfblk8/1 -> cfblk7/1
  cfblk7/1 -> cfblk4/1
  cfblk3/1 -> cfblk7/2
  cfblk10/1 -> cfblk8/1
  cfblk1/1 -> cfblk2/1

== system sampleModel1488/cfblk160/cfblk9 ==
  cfblk1 : Inport
  cfblk6 : Inport  Port=2
  cfblk7 : Inport  Port=3
  cfblk8 : Inport  Port=4
  cfblk3 : simulink/Discrete/Transfer Fcn First Order  PoleZ=0.95  ICPrevOutput=0.0  DoSatur=off
  cfblk4 : DiscreteFir  SampleTime=1
  cfblk5 : ComplexToMagnitudeAngle
  cfblk2 : Outport
  cfblk9 : Outport  Port=2
  wires:
  cfblk7/1 -> cfblk9/1
  cfblk8/1 -> cfblk4/1
  cfblk1/1 -> cfblk5/1
  cfblk4/1 -> cfblk2/1
  cfblk5/1 -> cfblk3/1

== system sampleModel1488/cfblk161/cfblk4 ==
  cfblk1 : Inport
  cfblk13 : Inport  Port=2
  cfblk14 : Inport  Port=3
  cfblk15 : Inport  Port=4
  cfblk10 : slpidlib/PID Controller (2DOF)  Controller=PID  Form=Parallel  TimeDomain=Discrete-time  UseExternalTs=off  SampleTime=1  IntegratorMethod=Forward Euler  FilterMethod=Forward Euler  ControllerParametersSource=internal  P=1  I=1  UseKiTs=off  D=0  N=100  UseFilter=on  b=1  c=1  TunerSelectOption=Transfer Function Based (PID Tuner App)  InitialConditionSource=internal  InitialConditionForIntegrator=0  InitialConditionForFilter=0  DifferentiatorICPrevScaledInput=0  ExternalReset=none  TrackingMode=off  Kt=1  LimitOutput=off  SatLimitsSource=internal  UpperSaturationLimit=inf  LowerSaturationLimit=-inf  LinearizeAsGain=off  AntiWindupMode=none  Kb=1  LimitIntegrator=off  UpperIntegratorSaturationLimit=inf  LowerIntegratorSaturationLimit=-inf  POutMin=[]  POutMax=[]  IOutMin=[]  IOutMax=[]  DOutMin=[]  DOutMax=[]  NOutMin=[]  NOutMax=[]  bOutMin=[]  bOutMax=[]  cOutMin=[]  cOutMax=[]  SumOutMin=[]  SumOutMax=[]  SaturationOutMin=[]  SaturationOutMax=[]  PParamMin=[]  PParamMax=[]  IParamMin=[]  IParamMax=[]  DParamMin=[]  DParamMax=[]  NParamMin=[]  NParamMax=[]  bParamMin=[]  bParamMax=[]  cParamMin=[]  cParamMax=[]  KbParamMin=[]  KbParamMax=[]  KtParamMin=[]  KtParamMax=[]  KbOutMin=[]  KbOutMax=[]  KtOutMin=[]  KtOutMax=[]  IntegratorOutMin=[]  IntegratorOutMax=[]  FilterOutMin=[]  FilterOutMax=[]  SumI1OutMin=[]  SumI1OutMax=[]  SumI2OutMin=[]  SumI2OutMax=[]  SumI3OutMin=[]  SumI3OutMax=[]  SumI4OutMin=[]  SumI4OutMax=[]  SumDOutMin=[]  SumDOutMax=[]  Sum1OutMin=[]  Sum1OutMax=[]  Sum2OutMin=[]  Sum2OutMax=[]  Sum3OutMin=[]  Sum3OutMax=[]  DifferentiatorOutMin=[]  DifferentiatorOutMax=[]  FilterDiffOutCoefMin=[]  FilterDiffOutCoefMax=[]  ReciprocalOutMin=[]  ReciprocalOutMax=[]  SumDenOutMin=[]  SumDenOutMax=[]  SumNumOutMin=[]  SumNumOutMax=[]  DivideOutMin=[]  DivideOutMax=[]  UdiffTsProdOutMin=[]  UdiffTsProdOutMax=[]  NTsProdOutMin=[]  NTsProdOutMax=[]  UintegralTsProdOutMin=[]  UintegralTsProdOutMax=[]  UngainTsProdOutMin=[]  UngainTsProdOutMax=[]  ClampingZeroOutDataTypeStr=Inherit: Inherit via back propagation  ClampingZeroOutMin=[]  ClampingZeroOutMax=[]  FilterDenConstantOutDataTypeStr=Inherit: Inherit via back propagation  FilterDenConstantOutMin=[]  FilterDenConstantOutMax=[]  PCopyOutDataTypeStr=Inherit: Inherit via back propagation  PCopyOutMin=[]  PCopyOutMax=[]  NCopyOutDataTypeStr=Inherit: Inherit via back propagation  NCopyOutMin=[]  NCopyOutMax=[]  IntegratorContinuousStateAttributes=''  IntegratorStateMustResolveToSignalObject=off  IntegratorRTWStateStorageClass=Auto  FilterContinuousStateAttributes=''  FilterStateMustResolveToSignalObject=off  FilterRTWStateStorageClass=Auto  ParallelPVariant=InternalParameters  IdealPVariant=Disabled  IVariant=InternalParameters  DVariant=InternalParameters  bVariant=InternalParameters  cVariant=InternalParameters  IntegratorVariant=Discrete  SatVariant=Disabled  AWVariant=Passthrough  PCopyVariant=Disabled  TRVariant=Disabled  FdbkBlocksVariant=Forward  IdealPFdbkVariant=Disabled  SatFdbkVariant=Disabled  DerivativeFilterVariant=ForwardEulerFilter  NVariant=InternalParameters  NCopyVariant=Disabled  FilterICVariant=InternalICsFilter  IntegratorICVariant=InternalICs  ExternalResetVariant=Disabled  TRSumVariant=Passthrough  SumFdbkVariant=Disabled  SumVariant=Sum_PID  TsampFilterVariant=InternalTs  TsampNgainVariant=Passthrough  TsampIntegralVariant=Disabled_SignalSpec  ExternalSaturationOutDataTypeStr=Inherit: Same as second input
      settings: LibrarySourceBlock=simulink/Discrete/Discrete PID Controller (2DOF)
  cfblk11 : simulink/Math Operations/MinMax Running Resettable  Function=min  vinit=0.0
  cfblk12 : ComplexToRealImag
  cfblk17 : Delay  SampleTime=1
  cfblk18 : Delay  SampleTime=1
  cfblk3 : DiscreteFilter  SampleTime=1
  cfblk4 : DiscreteStateSpace
  cfblk5 : DiscreteTransferFcn  SampleTime=1
  cfblk6 : simulink/Discrete/Difference  ICPrevInput=0.0  OutMin=[]  OutMax=[]  OutDataTypeStr=Inherit: Inherit via back propagation  OutDataType=fixdt(1, 16)  OutScaling=2^-10  DoSatur=off
  cfblk7 : simulink/Discrete/Transfer Fcn Lead or Lag  PoleZ=0.95  ZeroZ=0.75  ICPrevOutput=0.0  ICPrevInput=0.0  DoSatur=off
  cfblk8 : slpidlib/PID Controller (2DOF)  Controller=PID  Form=Parallel  TimeDomain=Discrete-time  UseExternalTs=off  SampleTime=1  IntegratorMethod=Forward Euler  FilterMethod=Forward Euler  ControllerParametersSource=internal  P=1  I=1  UseKiTs=off  D=0  N=100  UseFilter=on  b=1  c=1  TunerSelectOption=Transfer Function Based (PID Tuner App)  InitialConditionSource=internal  InitialConditionForIntegrator=0  InitialConditionForFilter=0  DifferentiatorICPrevScaledInput=0  ExternalReset=none  TrackingMode=off  Kt=1  LimitOutput=off  SatLimitsSource=internal  UpperSaturationLimit=inf  LowerSaturationLimit=-inf  LinearizeAsGain=off  AntiWindupMode=none  Kb=1  LimitIntegrator=off  UpperIntegratorSaturationLimit=inf  LowerIntegratorSaturationLimit=-inf  POutMin=[]  POutMax=[]  IOutMin=[]  IOutMax=[]  DOutMin=[]  DOutMax=[]  NOutMin=[]  NOutMax=[]  bOutMin=[]  bOutMax=[]  cOutMin=[]  cOutMax=[]  SumOutMin=[]  SumOutMax=[]  SaturationOutMin=[]  SaturationOutMax=[]  PParamMin=[]  PParamMax=[]  IParamMin=[]  IParamMax=[]  DParamMin=[]  DParamMax=[]  NParamMin=[]  NParamMax=[]  bParamMin=[]  bParamMax=[]  cParamMin=[]  cParamMax=[]  KbParamMin=[]  KbParamMax=[]  KtParamMin=[]  KtParamMax=[]  KbOutMin=[]  KbOutMax=[]  KtOutMin=[]  KtOutMax=[]  IntegratorOutMin=[]  IntegratorOutMax=[]  FilterOutMin=[]  FilterOutMax=[]  SumI1OutMin=[]  SumI1OutMax=[]  SumI2OutMin=[]  SumI2OutMax=[]  SumI3OutMin=[]  SumI3OutMax=[]  SumI4OutMin=[]  SumI4OutMax=[]  SumDOutMin=[]  SumDOutMax=[]  Sum1OutMin=[]  Sum1OutMax=[]  Sum2OutMin=[]  Sum2OutMax=[]  Sum3OutMin=[]  Sum3OutMax=[]  DifferentiatorOutMin=[]  DifferentiatorOutMax=[]  FilterDiffOutCoefMin=[]  FilterDiffOutCoefMax=[]  ReciprocalOutMin=[]  ReciprocalOutMax=[]  SumDenOutMin=[]  SumDenOutMax=[]  SumNumOutMin=[]  SumNumOutMax=[]  DivideOutMin=[]  DivideOutMax=[]  UdiffTsProdOutMin=[]  UdiffTsProdOutMax=[]  NTsProdOutMin=[]  NTsProdOutMax=[]  UintegralTsProdOutMin=[]  UintegralTsProdOutMax=[]  UngainTsProdOutMin=[]  UngainTsProdOutMax=[]  ClampingZeroOutDataTypeStr=Inherit: Inherit via back propagation  ClampingZeroOutMin=[]  ClampingZeroOutMax=[]  FilterDenConstantOutDataTypeStr=Inherit: Inherit via back propagation  FilterDenConstantOutMin=[]  FilterDenConstantOutMax=[]  PCopyOutDataTypeStr=Inherit: Inherit via back propagation  PCopyOutMin=[]  PCopyOutMax=[]  NCopyOutDataTypeStr=Inherit: Inherit via back propagation  NCopyOutMin=[]  NCopyOutMax=[]  IntegratorContinuousStateAttributes=''  IntegratorStateMustResolveToSignalObject=off  IntegratorRTWStateStorageClass=Auto  FilterContinuousStateAttributes=''  FilterStateMustResolveToSignalObject=off  FilterRTWStateStorageClass=Auto  ParallelPVariant=InternalParameters  IdealPVariant=Disabled  IVariant=InternalParameters  DVariant=InternalParameters  bVariant=InternalParameters  cVariant=InternalParameters  IntegratorVariant=Discrete  SatVariant=Disabled  AWVariant=Passthrough  PCopyVariant=Disabled  TRVariant=Disabled  FdbkBlocksVariant=Forward  IdealPFdbkVariant=Disabled  SatFdbkVariant=Disabled  DerivativeFilterVariant=ForwardEulerFilter  NVariant=InternalParameters  NCopyVariant=Disabled  FilterICVariant=InternalICsFilter  IntegratorICVariant=InternalICs  ExternalResetVariant=Disabled  TRSumVariant=Passthrough  SumFdbkVariant=Disabled  SumVariant=Sum_PID  TsampFilterVariant=InternalTs  TsampNgainVariant=Passthrough  TsampIntegralVariant=Disabled_SignalSpec  ExternalSaturationOutDataTypeStr=Inherit: Same as second input
      settings: LibrarySourceBlock=simulink/Discrete/Discrete PID Controller (2DOF)
  cfblk9 : DiscreteIntegrator  ICPrevOutput=DiscIntNeverNeededParam  ICPrevScaledInput=DiscIntNeverNeededParam
  cfblk2 : Outport
  cfblk16 : Outport  Port=2
  wires:
  cfblk7/1 -> cfblk4/1
  cfblk3/1 -> cfblk12/1
  cfblk13/1 -> cfblk11/1
  cfblk4/1 -> cfblk10/1
  cfblk8/1 -> cfblk10/2
  cfblk6/1 -> cfblk11/2
  cfblk12/1 -> cfblk5/1
  cfblk11/1 -> cfblk7/1
  cfblk9/1 -> cfblk16/1
  cfblk15/1 -> cfblk2/1
  cfblk5/1 -> cfblk6/1
  cfblk14/1 -> cfblk9/1
  cfblk1/1 -> cfblk8/2
  cfblk10/1 -> cfblk17/1
  cfblk17/1 -> cfblk8/1
  cfblk12/2 -> cfblk18/1
  cfblk18/1 -> cfblk3/1

== system sampleModel1488/cfblk161/cfblk5 ==
  cfblk1 : Inport
  cfblk7 : Inport  Port=2
  cfblk8 : Inport  Port=3
  cfblk3 : simulink/Discrete/Transfer Fcn First Order  PoleZ=0.95  ICPrevOutput=0.0  DoSatur=off
  cfblk4 : simulink/Discrete/Transfer Fcn First Order  PoleZ=0.95  ICPrevOutput=0.0  DoSatur=off
  cfblk5 : Sin  TimeSource=Use external signal  SampleTime=0
  cfblk6 : Constant  Value=[140778174.315885]  SampleTime=1
  cfblk2 : Outport
  cfblk9 : Outport  Port=2
  cfblk10 : Outport  Port=3
  wires:
  cfblk8/1 -> cfblk2/1
  cfblk4/1 -> cfblk9/1
  cfblk7/1 -> cfblk3/1
  cfblk5/1 -> cfblk4/1
  cfblk3/1 -> cfblk5/1
  cfblk1/1 -> cfblk10/1

== system sampleModel1488/cfblk162/cfblk7 ==
  cfblk1 : Inport
  cfblk11 : Inport  Port=2
  cfblk12 : Inport  Port=3
  cfblk13 : Inport  Port=4
  cfblk14 : Inport  Port=5
  cfblk15 : Inport  Port=6
  cfblk10 : Constant  Value=[29253716.620342]  SampleTime=1
  cfblk3 : UnitDelay  HasFrameUpgradeWarning=on
  cfblk4 : simulink/Discrete/Difference  ICPrevInput=0.0  OutMin=[]  OutMax=[]  OutDataTypeStr=Inherit: Inherit via back propagation  OutDataType=fixdt(1, 16)  OutScaling=2^-10  DoSatur=off
  cfblk5 : UnitDelay  HasFrameUpgradeWarning=on
  cfblk6 : Delay  DelayLengthSource=Input port  SampleTime=1
      settings: InputPortMap=u0,p1
  cfblk7 : DiscreteFir  SampleTime=1
  cfblk8 : Sum  Inputs=+-
  cfblk9 : Signum
  cfblk2 : Outport
  wires:
  cfblk10/1 -> cfblk3/1
  cfblk6/1 -> cfblk2/1
  cfblk12/1 -> cfblk7/1
  cfblk3/1 -> cfblk4/1
  cfblk9/1 -> cfblk8/1
  cfblk1/1 -> cfblk5/1
  cfblk4/1 -> cfblk6/1
  cfblk15/1 -> cfblk9/1
  cfblk5/1 -> cfblk8/2
  cfblk14/1 -> cfblk6/2

== system sampleModel1488/cfblk162/cfblk8 ==
  cfblk1 : Inport
  cfblk6 : Inport  Port=2
  cfblk3 : Sum  Inputs=+
  cfblk4 : Trigonometry
  cfblk5 : Constant  Value=[870557979.746877]  SampleTime=1
  cfblk2 : Outport
  cfblk7 : Outport  Port=2
  wires:
  cfblk1/1 -> cfblk4/1
  cfblk4/1 -> cfblk7/1
  cfblk5/1 -> cfblk2/1
  cfblk6/1 -> cfblk3/1

== system sampleModel1488/cfblk164/cfblk10 ==
  cfblk1 : Inport
  cfblk10 : Inport  Port=2
  cfblk11 : Inport  Port=3
  Action Port : ActionPort  ActionPortLabel=else
  cfblk13 : Delay
  cfblk3 : Delay
  cfblk4 : Sqrt  Operator=rSqrt  AlgorithmType=Newton-Raphson
  cfblk5 : Trigonometry
  cfblk6 : Squeeze
  cfblk7 : Sum  Inputs=+
  cfblk8 : Sum  Inputs=+-
  cfblk9 : Reshape
  cfblk2 : Outport
  cfblk12 : Outport  Port=2
  wires:
  cfblk11/1 -> cfblk7/1
  cfblk10/1 -> cfblk6/1
  cfblk4/1 -> cfblk12/1
  cfblk7/1 -> cfblk9/1
  cfblk8/1 -> cfblk4/1
  cfblk6/1 -> cfblk2/1
  cfblk1/1 -> cfblk8/1
  cfblk9/1 -> cfblk8/2
  cfblk3/1 -> cfblk5/1
  cfblk5/1 -> cfblk13/1
  cfblk13/1 -> cfblk3/1

== system sampleModel1488/cfblk164/cfblk5 ==
  cfblk1 : Inport
  cfblk8 : Inport  Port=2
  cfblk3 : simulink/Discrete/Transfer Fcn Lead or Lag  PoleZ=0.95  ZeroZ=0.75  ICPrevOutput=0.0  ICPrevInput=0.0  DoSatur=off
  cfblk4 : Signum
  cfblk5 : Sqrt
  cfblk6 : Abs  SaturateOnIntegerOverflow=off
  cfblk7 : Constant  Value=[-65404291.431518]  SampleTime=1
  cfblk2 : Outport
  wires:
  cfblk3/1 -> cfblk6/1
  cfblk1/1 -> cfblk3/1
  cfblk7/1 -> cfblk2/1
  cfblk6/1 -> cfblk5/1
  cfblk8/1 -> cfblk4/1

== system sampleModel1488/cfblk164/cfblk6 ==
  cfblk1 : Inport
  cfblk15 : Inport  Port=2
  cfblk10 : Sin  TimeSource=Use external signal  SampleTime=0
  cfblk11 : Sqrt  Operator=rSqrt  AlgorithmType=Newton-Raphson
  cfblk12 : simulink/Math Operations/Slider Gain  gain=1  low=0  high=2
  cfblk13 : UnaryMinus
  cfblk14 : simulink/Math Operations/Slider Gain  gain=1  low=0  high=2
  cfblk18 : Delay  SampleTime=1
  cfblk3 : DiscreteFilter  SampleTime=1
  cfblk4 : DiscreteFir  SampleTime=1
  cfblk5 : DiscreteTransferFcn  SampleTime=1
  cfblk6 : slpidlib/PID Controller (2DOF)  Controller=PID  Form=Parallel  TimeDomain=Discrete-time  UseExternalTs=off  SampleTime=1  IntegratorMethod=Forward Euler  FilterMethod=Forward Euler  ControllerParametersSource=internal  P=1  I=1  UseKiTs=off  D=0  N=100  UseFilter=on  b=1  c=1  TunerSelectOption=Transfer Function Based (PID Tuner App)  InitialConditionSource=internal  InitialConditionForIntegrator=0  InitialConditionForFilter=0  DifferentiatorICPrevScaledInput=0  ExternalReset=none  TrackingMode=off  Kt=1  LimitOutput=off  SatLimitsSource=internal  UpperSaturationLimit=inf  LowerSaturationLimit=-inf  LinearizeAsGain=off  AntiWindupMode=none  Kb=1  LimitIntegrator=off  UpperIntegratorSaturationLimit=inf  LowerIntegratorSaturationLimit=-inf  POutMin=[]  POutMax=[]  IOutMin=[]  IOutMax=[]  DOutMin=[]  DOutMax=[]  NOutMin=[]  NOutMax=[]  bOutMin=[]  bOutMax=[]  cOutMin=[]  cOutMax=[]  SumOutMin=[]  SumOutMax=[]  SaturationOutMin=[]  SaturationOutMax=[]  PParamMin=[]  PParamMax=[]  IParamMin=[]  IParamMax=[]  DParamMin=[]  DParamMax=[]  NParamMin=[]  NParamMax=[]  bParamMin=[]  bParamMax=[]  cParamMin=[]  cParamMax=[]  KbParamMin=[]  KbParamMax=[]  KtParamMin=[]  KtParamMax=[]  KbOutMin=[]  KbOutMax=[]  KtOutMin=[]  KtOutMax=[]  IntegratorOutMin=[]  IntegratorOutMax=[]  FilterOutMin=[]  FilterOutMax=[]  SumI1OutMin=[]  SumI1OutMax=[]  SumI2OutMin=[]  SumI2OutMax=[]  SumI3OutMin=[]  SumI3OutMax=[]  SumI4OutMin=[]  SumI4OutMax=[]  SumDOutMin=[]  SumDOutMax=[]  Sum1OutMin=[]  Sum1OutMax=[]  Sum2OutMin=[]  Sum2OutMax=[]  Sum3OutMin=[]  Sum3OutMax=[]  DifferentiatorOutMin=[]  DifferentiatorOutMax=[]  FilterDiffOutCoefMin=[]  FilterDiffOutCoefMax=[]  ReciprocalOutMin=[]  ReciprocalOutMax=[]  SumDenOutMin=[]  SumDenOutMax=[]  SumNumOutMin=[]  SumNumOutMax=[]  DivideOutMin=[]  DivideOutMax=[]  UdiffTsProdOutMin=[]  UdiffTsProdOutMax=[]  NTsProdOutMin=[]  NTsProdOutMax=[]  UintegralTsProdOutMin=[]  UintegralTsProdOutMax=[]  UngainTsProdOutMin=[]  UngainTsProdOutMax=[]  ClampingZeroOutDataTypeStr=Inherit: Inherit via back propagation  ClampingZeroOutMin=[]  ClampingZeroOutMax=[]  FilterDenConstantOutDataTypeStr=Inherit: Inherit via back propagation  FilterDenConstantOutMin=[]  FilterDenConstantOutMax=[]  PCopyOutDataTypeStr=Inherit: Inherit via back propagation  PCopyOutMin=[]  PCopyOutMax=[]  NCopyOutDataTypeStr=Inherit: Inherit via back propagation  NCopyOutMin=[]  NCopyOutMax=[]  IntegratorContinuousStateAttributes=''  IntegratorStateMustResolveToSignalObject=off  IntegratorRTWStateStorageClass=Auto  FilterContinuousStateAttributes=''  FilterStateMustResolveToSignalObject=off  FilterRTWStateStorageClass=Auto  ParallelPVariant=InternalParameters  IdealPVariant=Disabled  IVariant=InternalParameters  DVariant=InternalParameters  bVariant=InternalParameters  cVariant=InternalParameters  IntegratorVariant=Discrete  SatVariant=Disabled  AWVariant=Passthrough  PCopyVariant=Disabled  TRVariant=Disabled  FdbkBlocksVariant=Forward  IdealPFdbkVariant=Disabled  SatFdbkVariant=Disabled  DerivativeFilterVariant=ForwardEulerFilter  NVariant=InternalParameters  NCopyVariant=Disabled  FilterICVariant=InternalICsFilter  IntegratorICVariant=InternalICs  ExternalResetVariant=Disabled  TRSumVariant=Passthrough  SumFdbkVariant=Disabled  SumVariant=Sum_PID  TsampFilterVariant=InternalTs  TsampNgainVariant=Passthrough  TsampIntegralVariant=Disabled_SignalSpec  ExternalSaturationOutDataTypeStr=Inherit: Same as second input
      settings: LibrarySourceBlock=simulink/Discrete/Discrete PID Controller (2DOF)
  cfblk7 : Product  Inputs=*
  cfblk8 : Trigonometry
  cfblk9 : Product
  cfblk2 : Outport
  cfblk16 : Outport  Port=2
  cfblk17 : Outport  Port=3
  wires:
  cfblk14/1 -> cfblk17/1
  cfblk15/1 -> cfblk8/1, cfblk6/2
  cfblk8/1 -> cfblk5/1
  cfblk12/1 -> cfblk14/1
  cfblk6/1 -> cfblk7/1, cfblk13/1
  cfblk4/1 -> cfblk10/1
  cfblk5/1 -> cfblk9/1
  cfblk13/1 -> cfblk11/1
  cfblk10/1 -> cfblk16/1
  cfblk1/1 -> cfblk12/1, cfblk4/1
  cfblk11/1 -> cfblk2/1
  cfblk3/1 -> cfblk6/1
  cfblk7/1 -> cfblk9/2
  cfblk9/1 -> cfblk18/1
  cfblk18/1 -> cfblk3/1

== system sampleModel1488/cfblk164/cfblk9 ==
  cfblk1 : Inport
  cfblk12 : Inport  Port=2
  cfblk13 : Inport  Port=3
  cfblk14 : Inport  Port=4
  Action Port : ActionPort  ActionPortLabel=if(u1 >= 0)
  cfblk10 : Constant  Value=[856839119.245301]  SampleTime=1
  cfblk11 : Constant  Value=[-443879876.454567]  SampleTime=1
  cfblk3 : simulink/Discrete/Transfer Fcn Real Zero  ZeroZ=0.75  ICPrevInput=0.0  DoSatur=off
  cfblk4 : Signum
  cfblk5 : Signum
  cfblk6 : Constant  Value=[793891528.618960]  SampleTime=1
  cfblk7 : Constant  Value=[-416536826.113714]  SampleTime=1
  cfblk8 : Constant  Value=[-887411711.949198]  SampleTime=1
  cfblk9 : Constant  Value=[1195139.391758]  SampleTime=1
  cfblk2 : Outport
  cfblk15 : Outport  Port=2
  wires:
  cfblk12/1 -> cfblk4/1
  cfblk11/1 -> cfblk3/1
  cfblk10/1 -> cfblk15/1
  cfblk3/1 -> cfblk5/1
  cfblk8/1 -> cfblk2/1

== system sampleModel1488/cfblk165/cfblk6 ==
  cfblk1 : Inport
  cfblk11 : Inport  Port=2
  cfblk12 : Inport  Port=3
  cfblk13 : Inport  Port=4
  cfblk14 : Inport  Port=5
  cfblk10 : Constant  Value=[388771791.509372]  SampleTime=1
  cfblk16 : Delay  SampleTime=1
  cfblk3 : DiscreteFilter  SampleTime=1
  cfblk4 : simulink/Discrete/Transfer Fcn Lead or Lag  PoleZ=0.95  ZeroZ=0.75  ICPrevOutput=0.0  ICPrevInput=0.0  DoSatur=off
  cfblk5 : DiscreteFir  SampleTime=1
  cfblk6 : Product  Inputs=**
  cfblk7 : DotProduct  OutDataTypeStr=Inherit: Inherit via internal rule
  cfblk8 : MinMax  Function=max  Inputs=2
  cfblk9 : Trigonometry
  cfblk2 : Outport
  cfblk15 : Outport  Port=2
  wires:
  cfblk11/1 -> cfblk7/1
  cfblk7/1 -> cfblk5/1
  cfblk12/1 -> cfblk2/1
  cfblk1/1 -> cfblk9/1
  cfblk6/1 -> cfblk7/2
  cfblk5/1 -> cfblk8/1
  cfblk4/1 -> cfblk6/1
  cfblk3/1 -> cfblk4/1
  cfblk14/1 -> cfblk6/2
  cfblk10/1 -> cfblk8/2
  cfblk13/1 -> cfblk15/1
  cfblk8/1 -> cfblk16/1
  cfblk16/1 -> cfblk3/1

== system sampleModel1488/cfblk165/cfblk7 ==
  cfblk1 : Inport
  cfblk13 : Inport  Port=2
  cfblk10 : simulink/Math Operations/Slider Gain  gain=1  low=0  high=2
  cfblk11 : Constant  Value=[-609991204.218523]  SampleTime=1
  cfblk12 : Constant  Value=[-968827494.028482]  SampleTime=1
  cfblk15 : Delay  SampleTime=1
  cfblk3 : UnitDelay  HasFrameUpgradeWarning=on
  cfblk4 : slpidlib/PID Controller (2DOF)  Controller=PID  Form=Parallel  TimeDomain=Discrete-time  UseExternalTs=off  SampleTime=1  IntegratorMethod=Forward Euler  FilterMethod=Forward Euler  ControllerParametersSource=internal  P=1  I=1  UseKiTs=off  D=0  N=100  UseFilter=on  b=1  c=1  TunerSelectOption=Transfer Function Based (PID Tuner App)  InitialConditionSource=internal  InitialConditionForIntegrator=0  InitialConditionForFilter=0  DifferentiatorICPrevScaledInput=0  ExternalReset=none  TrackingMode=off  Kt=1  LimitOutput=off  SatLimitsSource=internal  UpperSaturationLimit=inf  LowerSaturationLimit=-inf  LinearizeAsGain=off  AntiWindupMode=none  Kb=1  LimitIntegrator=off  UpperIntegratorSaturationLimit=inf  LowerIntegratorSaturationLimit=-inf  POutMin=[]  POutMax=[]  IOutMin=[]  IOutMax=[]  DOutMin=[]  DOutMax=[]  NOutMin=[]  NOutMax=[]  bOutMin=[]  bOutMax=[]  cOutMin=[]  cOutMax=[]  SumOutMin=[]  SumOutMax=[]  SaturationOutMin=[]  SaturationOutMax=[]  PParamMin=[]  PParamMax=[]  IParamMin=[]  IParamMax=[]  DParamMin=[]  DParamMax=[]  NParamMin=[]  NParamMax=[]  bParamMin=[]  bParamMax=[]  cParamMin=[]  cParamMax=[]  KbParamMin=[]  KbParamMax=[]  KtParamMin=[]  KtParamMax=[]  KbOutMin=[]  KbOutMax=[]  KtOutMin=[]  KtOutMax=[]  IntegratorOutMin=[]  IntegratorOutMax=[]  FilterOutMin=[]  FilterOutMax=[]  SumI1OutMin=[]  SumI1OutMax=[]  SumI2OutMin=[]  SumI2OutMax=[]  SumI3OutMin=[]  SumI3OutMax=[]  SumI4OutMin=[]  SumI4OutMax=[]  SumDOutMin=[]  SumDOutMax=[]  Sum1OutMin=[]  Sum1OutMax=[]  Sum2OutMin=[]  Sum2OutMax=[]  Sum3OutMin=[]  Sum3OutMax=[]  DifferentiatorOutMin=[]  DifferentiatorOutMax=[]  FilterDiffOutCoefMin=[]  FilterDiffOutCoefMax=[]  ReciprocalOutMin=[]  ReciprocalOutMax=[]  SumDenOutMin=[]  SumDenOutMax=[]  SumNumOutMin=[]  SumNumOutMax=[]  DivideOutMin=[]  DivideOutMax=[]  UdiffTsProdOutMin=[]  UdiffTsProdOutMax=[]  NTsProdOutMin=[]  NTsProdOutMax=[]  UintegralTsProdOutMin=[]  UintegralTsProdOutMax=[]  UngainTsProdOutMin=[]  UngainTsProdOutMax=[]  ClampingZeroOutDataTypeStr=Inherit: Inherit via back propagation  ClampingZeroOutMin=[]  ClampingZeroOutMax=[]  FilterDenConstantOutDataTypeStr=Inherit: Inherit via back propagation  FilterDenConstantOutMin=[]  FilterDenConstantOutMax=[]  PCopyOutDataTypeStr=Inherit: Inherit via back propagation  PCopyOutMin=[]  PCopyOutMax=[]  NCopyOutDataTypeStr=Inherit: Inherit via back propagation  NCopyOutMin=[]  NCopyOutMax=[]  IntegratorContinuousStateAttributes=''  IntegratorStateMustResolveToSignalObject=off  IntegratorRTWStateStorageClass=Auto  FilterContinuousStateAttributes=''  FilterStateMustResolveToSignalObject=off  FilterRTWStateStorageClass=Auto  ParallelPVariant=InternalParameters  IdealPVariant=Disabled  IVariant=InternalParameters  DVariant=InternalParameters  bVariant=InternalParameters  cVariant=InternalParameters  IntegratorVariant=Discrete  SatVariant=Disabled  AWVariant=Passthrough  PCopyVariant=Disabled  TRVariant=Disabled  FdbkBlocksVariant=Forward  IdealPFdbkVariant=Disabled  SatFdbkVariant=Disabled  DerivativeFilterVariant=ForwardEulerFilter  NVariant=InternalParameters  NCopyVariant=Disabled  FilterICVariant=InternalICsFilter  IntegratorICVariant=InternalICs  ExternalResetVariant=Disabled  TRSumVariant=Passthrough  SumFdbkVariant=Disabled  SumVariant=Sum_PID  TsampFilterVariant=InternalTs  TsampNgainVariant=Passthrough  TsampIntegralVariant=Disabled_SignalSpec  ExternalSaturationOutDataTypeStr=Inherit: Same as second input
      settings: LibrarySourceBlock=simulink/Discrete/Discrete PID Controller (2DOF)
  cfblk5 : Delay  DelayLengthSource=Input port  SampleTime=1
      settings: InputPortMap=u0,p1
  cfblk6 : Bias  Bias=[-648749549.423812]  SaturateOnIntegerOverflow=off
  cfblk7 : Signum
  cfblk8 : Sin  TimeSource=Use external signal  SampleTime=0
  cfblk9 : Reshape
  cfblk2 : Outport
  cfblk14 : Outport  Port=2
  wires:
  cfblk12/1 -> cfblk9/1
  cfblk13/1 -> cfblk14/1
  cfblk9/1 -> cfblk6/1
  cfblk11/1 -> cfblk10/1
  cfblk4/1 -> cfblk8/1
  cfblk7/1 -> cfblk5/1
  cfblk8/1 -> cfblk7/1
  cfblk6/1 -> cfblk5/2
  cfblk10/1 -> cfblk3/1
  cfblk1/1 -> cfblk2/1
  cfblk3/1 -> cfblk4/2
  cfblk5/1 -> cfblk15/1
  cfblk15/1 -> cfblk4/1

== system sampleModel1488/cfblk165/cfblk8 ==
  cfblk1 : Inport
  cfblk11 : Inport  Port=2
  cfblk12 : Inport  Port=3
  cfblk13 : Inport  Port=4
  cfblk14 : Inport  Port=5
  cfblk15 : Inport  Port=6
  cfblk10 : Constant  Value=[-200088241.921868]  SampleTime=1
  cfblk17 : Delay  SampleTime=1
  cfblk3 : Delay  DelayLengthSource=Input port  SampleTime=1
      settings: InputPortMap=u0,p1
  cfblk4 : ComplexToMagnitudeAngle
  cfblk5 : Squeeze
  cfblk6 : DotProduct  OutDataTypeStr=Inherit: Inherit via internal rule
  cfblk7 : Product  Inputs=*
  cfblk8 : PermuteDimensions
  cfblk9 : Sum  Inputs=+-
  cfblk2 : Outport
  cfblk16 : Outport  Port=2
  wires:
  cfblk13/1 -> cfblk3/1
  cfblk10/1 -> cfblk8/1
  cfblk9/1 -> cfblk2/1
  cfblk15/1 -> cfblk9/1
  cfblk1/1 -> cfblk6/1
  cfblk14/1 -> cfblk4/1
  cfblk12/1 -> cfblk9/2
  cfblk4/1 -> cfblk3/2
  cfblk11/1 -> cfblk16/1
  cfblk5/1 -> cfblk7/1
  cfblk6/1 -> cfblk5/1
  cfblk7/1 -> cfblk17/1
  cfblk17/1 -> cfblk6/2
